simulink model "HEV_SeriesParallel"  (R2022b)
settings: Solver=ode23t  StartTime=0.0  StopTime=100  RelTol=0.0001  AbsTol=1e-05  EnableMultiTasking=on
PreLoadFcn:
  | load UrbanCycle1
  | load UrbanCycle2
  | load UrbanCycle3
  | load UrbanCycle4
  | load UrbanCycle5
  | 
  | assignin('base','decimation',1)
  | Pbatt = 21e3;
  | Vbatt =100;
  | Ts = 6e-5;   % time step
  | 
  | Drive_Cycle_Num = 1;
  | warning off Simulink:Commands:LoadMdlParameterizedLink
PostLoadFcn:
  | warning off Simulink:Engine:UsingDefaultMaxStepSize
  | warning off Simulink:blocks:MatchingGotoNotFound
  | warning off Simulink:blocks:MatchingFromNotFound
  | warning off Simulink:blocks:TDelayBufferTooSmall
  | warning off Simulink:SL_SaveWithParameterizedLinks_Warning
  | warning off Simulink:SL_TDelayBufferTooSmall
  | warning off Simulink:SL_OutputNotConnected
  | warning off Simulink:SL_SaveWithDisabledLinks_Warning
  | 
  | warning off Simulink:SL_SetParamLinkChangeWarn
  | 
  | warning('off','Simulink:SL_UINotUpdatedDuringRapidAccelSim');
  | warning off Simulink:Engine:OutputNotConnected
  | warning off Simulink:Engine:UINotUpdatedDuringRapidAccelSim
  | warning off Simulink:Engine:SaveWithParameterizedLinks_Warning
  | warning off Simulink:Engine:SolverMaskedZC
  | set_param('HEV_SeriesParallel','MaskedZcDiagnostic','none');
  | warning off Simulink:Engine:SolverInconsistentInitialConditionsWarnForDAE
  | set_param('HEV_SeriesParallel','IgnoredZcDiagnostic','none');
  | warning off Simulink:Engine:SolverIgnoredZCBracketing
  | set_param('HEV_SeriesParallel','MaxConsecutiveZCsMsg','none');
  | warning off Simulink:Engine:SolverConsecutiveZCNum
  | warning off Simulink:Engine:SolverMinStepSizeWarnForDAE
  | warning off Simulink:Engine:SolverMinStepNonlinearIterWarnForDAE
  | warning off simscape:compiler:sli:init:SolverNotRecommended
  | warning off Simulink:Commands:SetParamLinkChangeWarn
  | warning off xPCTarget:sampleTime:sampleTimeInvariance
  | warning off Simulink:blocks:TDelayFixedBuffer
  | 
  | warning('off','physmod:common:gl:sli:rtp:InvalidNonValueReference')
  | warning('off','physmod:common:gl:sli:rtp:InvalidNonValueReferenceMask')
  | 
  | Setup_HEV_Model_Configurations
  | 
  | % Commands to avoid warning at first run
  | % PS battery function
  | warning off MATLAB:illConditionedMatrix
  | try
  |    set_param(bdroot, 'SimulationCommand', 'update');
  | catch
  | end
  | warning on MATLAB:illConditionedMatrix
InitFcn:
  | Configure_HEV_Simulation
StartFcn:
  | tic;
StopFcn:
  | Elapsed_Sim_Time = toc; disp(['Elapsed time for ' bdroot ' = ' num2str(Elapsed_Sim_Time)])
model workspace (MAT data in the model file):
  guiH = 18054.0001221
undefined symbols (not defined in the file or in its folder): HEV_Param, sigbuilder_block
libraries: fl_lib x18, nesl_utility x11, HEV_Electrical_Lib x3, sdl_lib x2, HEV_Vehicle_Dynamics_Lib x2, simulink x1, spspowerguiLib x1
(part 1 of 2)
Description:
  | Hybrid Electric Vehicle, Series-Parallel
  | 
  | Copyright 2014-2022 The MathWorks(TM), Inc.
settings Model: ExtModeTrigDuration=200  TunableVars=Drive_Cycle_Num  TunableVarsStorageClass=Auto  Creator=tegel  LastModifiedBy=fedformi_new
settings SolverCC: AutoScaleAbsTol=off  ZcThreshold=0  ConsecutiveZCsStepRelTol=0.0001  ConcurrentTasks=on  ZeroCrossAlgorithm=Adaptive  AlgebraicLoopSolver=TrustRegion  PositivePriorityOrder=on
settings DataIOCC: SaveFormat=Array  SignalLoggingSaveFormat=ModelDataLogs  SignalLogging=off  DSMLogging=off  ReturnWorkspaceOutputs=off
settings OptimizationCC: BlockReduction=off  OptimizeBlockIOStorage=off  BufferReuse=off  GlobalBufferReuse=off  ExpressionFolding=off  ExpressionDepthLimit=2147483647  LocalBlockOutputs=off  ZeroExternalMemoryAtStartup=off  ZeroInternalMemoryAtStartup=off  InitFltsAndDblsToZero=on  EfficientMapNaN2IntZero=off  OptimizeDataStoreBuffers=off  BusAssignmentInplaceUpdate=off
settings DebuggingCC: AlgebraicLoopMsg=error  UnderspecifiedInitializationDetection=Classic  MergeDetectMultiDrivingBlocksExec=none  SignalResolutionControl=TryResolveAllWithWarning  MaxConsecutiveZCsMsg=none  MaskedZcDiagnostic=none  IgnoredZcDiagnostic=none  SigSpecEnsureSampleTimeMsg=none  FcnCallInpInsideContextMsg=warning  UnconnectedInputMsg=warning  UnconnectedOutputMsg=warning  UnconnectedLineMsg=warning  AllowSymbolicDim=off  UnknownTsInhSupMsg=none  StateNameClashWarn=warning  PregeneratedLibrarySubsystemCodeDiagnostic=none  SFUnexpectedBacktrackingDiag=warning  SFNoUnconditionalDefaultTransitionDiag=warning  SFExecutionAtInitializationDiag=none  SFMachineParentedDataDiag=warning  ArithmeticOperatorsInVariantConditions=warning
settings HardwareCC: TargetBitPerLong=64  TargetBitPerPointer=64  TargetBitPerSizeT=64  TargetBitPerPtrDiffT=64  TargetLongLongMode=on  TargetIntDivRoundTo=Zero  TargetEndianess=LittleEndian  TargetWordSize=64  TargetHWDeviceType=MATLAB Host
settings ModelReferenceCC: EnableRefExpFcnMdlSchedulingChecks=on  PropagateSignalLabelsOutOfModel=off
settings SFSimCC: SimUseLocalCustomCode=off  SimParseCustomCode=off  CustomCodeUndefinedFunction=UseInterfaceOnly
settings RTWCC: RTWUseLocalCustomCode=off  Toolchain=Simulink Real-Time Toolchain  BuildConfiguration=Faster Runs  TargetLang=C++  DLArmComputeVersion=19.05
settings CodeAppCC: StateflowObjectComments=on
settings GRTTargetCC: TargetLangStandard=C++03 (ISO)  CodeInterfacePackaging=C++ class
settings ConfigComp: CovMetricSettings=dw  CovSaveCumulativeToWorkspaceVar=on  CovSaveSingleToWorkspaceVar=on  CovExternalEMLEnable=off  CovSFcnEnable=off
settings SimscapeCC: ExplicitSolverDiagnosticOptions=none  SimscapeNormalizeSystem=off  SimscapeLogType=all  SimscapeLogName=simlog_HEVSP  SimscapeLogLimitData=off

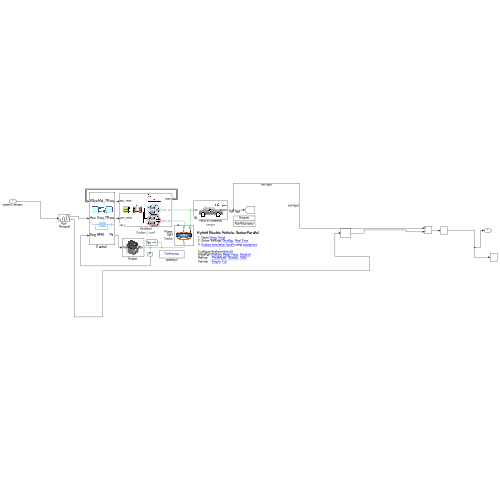
[thumbnail: Simulink's stored preview of the top-level diagram]
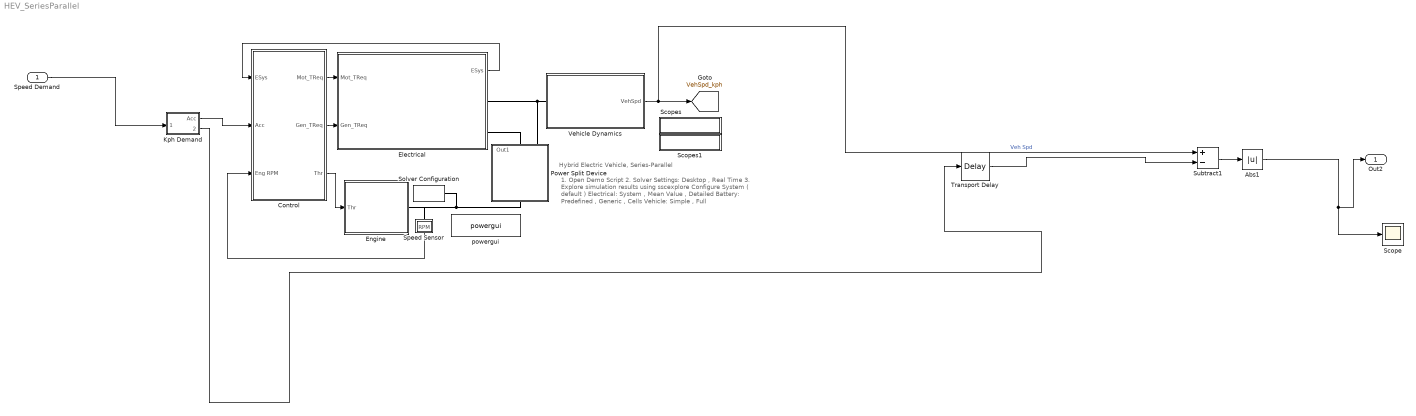
== system HEV_SeriesParallel ==
  note: 1. Open Demo Script
      | 2. Solver Settings: Desktop , Real Time
      | 3. Explore simulation results using sscexplore
      |
      | Configure System ( default )
      | Electrical: System , Mean Value , Detailed
      | Battery: Predefined , Generic , Cells
      | Vehicle: Simple , Full
  note: Hybrid Electric Vehicle, Series-Parallel
  Speed Demand : Inport
  Abs1 : Abs  SaturateOnIntegerOverflow=off
  Control : Subsystem
      mask Display:
      | image('HEV_Control_IMAGE.jpg');
      | port_label('input',1,'ESys');
      | port_label('input',2,'Acc');
      | port_label('input',3,'Eng RPM');
      | port_label('output',1,'Mot_TReq');
      | port_label('output',2,'Gen_TReq');
      | port_label('output',3,'Thr');
  Electrical : Subsystem  BlockChoice=System Level  Variant=on  VariantControlMode=label  LabelModeActiveChoice=System_Level  mask{popup_electricalvariant=System Level, popup_batteryvariantsystem=Predefined, popup_batteryvariantdetailed=Generic}
      mask prompts: popup_electricalvariant "Fidelity of Electrical System"; popup_batteryvariantsystem "Battery Model"; popup_batteryvariantdetailed "Battery Model"
      mask init:
      | if(popup_electricalvariant==1)
      |     set_param(gcb,'LabelModeActiveChoice','System_Level');
      |     set_param([gcb '/System Level'],'popup_batteryvariant',get_param(gcb,'popup_batteryvariantsystem'));
      | elseif(popup_electricalvariant==2)
      | 	set_param(gcb,'LabelModeActiveChoice','Mean_Value');
      |     set_param([gcb '/Mean Value'],'popup_batteryvariant',get_param(gcb,'popup_batteryvariantdetailed'));
      | elseif(popup_electricalvariant==3)
      |     set_param(gcb,'LabelModeActiveChoice','Detailed');
      |     set_param([gcb '/Detailed'],'popup_batteryvariant',get_param(gcb,'popup_batteryvariantdetailed'));
      | end
      | 
      | %blk = find_system(gcbh, 'FollowLinks','on','SearchDepth', 1, 'Parent', gcb, 'VariantObject', get_param(gcb,'activevariant'));
      settings: AttributesFormatString=%<ActiveVariant>
      mask TypeOptions popup_electricalvariant: System Level | Mean Value | Detailed
      mask Callback popup_electricalvariant:
      | maskObj = Simulink.Mask.get(gcb);
      | bas_h = maskObj.getParameter('popup_batteryvariantsystem');
      | bad_h = maskObj.getParameter('popup_batteryvariantdetailed');
      | if strcmp(get_param(gcb,'popup_electricalvariant'),'System Level')
      |     bas_h.Visible = 'on';
      |     bad_h.Visible = 'off';
      | else
      |     bas_h.Visible = 'off';
      |     bad_h.Visible = 'on';
      | end
      | clear maskObj
      mask TypeOptions popup_batteryvariantsystem: Predefined | Generic | Cells
      mask TypeOptions popup_batteryvariantdetailed: Predefined | Generic
      mask Display:
      | ele_var = get_param(gcb,'ActiveVariant');
      | batt_var = get_param([gcb '/' strrep(ele_var,'_',' ') '/Battery'],'ActiveVariant');
      | imagestr = ['HEV_Electrical_' strrep(ele_var,'_','') '_' batt_var '_IMAGE.jpg'];
      | image(imagestr);
  Engine : Subsystem  RequirementInfo={} %GIDa_8d15d6ea_be00_49db_a7ed_57a5c222ce3a
      mask Display:
      | image('HEV_Engine_IMAGE.jpg');
      | port_label('input',1,'Thr');
      | port_label('RConn',1,'Sh');
  Kph Demand : Subsystem
      mask Display:
      | plotstr=['UrbanCycle' evalin('base','num2str(Drive_Cycle_Num)')];
      | plot(evalin('base',[plotstr '.time']),evalin('base',[plotstr '.SpdKph']));
      | text(evalin('base',['0.7*max(' plotstr '.time)']),evalin('base',['0.25*max(' plotstr '.SpdKph)']),evalin('base','num2str(Drive_Cycle_Num)'));
  Power Split Device : Subsystem
      mask Display:
      | image('HEV_Planetary_Gear_IMAGE.jpg');
      | color('black');
      | port_label('Lconn',1,'C');
      | port_label('Rconn',1,'S');
      | port_label('Rconn',2,'R');
  Scope : Scope
  Scopes : Subsystem  mask(Data Acquisition){}
      mask Display: disp('Scopes');
  Scopes1 : Subsystem  mask(Data Acquisition){}
      mask Display: disp('Fuel Economy');
  Solver Configuration : nesl_utility/Solver Configuration  PhysicalDomain=network_engine_domain  SubClassName=solver  LeftPortType=input  RightPortType=generic  Tones=[]  Harmonics=[]  SimulateNoise=off  Profile=off  UseLocalSampling=off  EnableSwitchedLinearOptims=on  FrequencyDomain=off  UseCCode=off  RelTol=0.001  AbsTol=1e-06  MinStep=1e-09  ToWorkspace=off  RevertToSquareIcSolve=off  NumHomotopyIterations=100  PhasorMode=off  PhasorModeNumHarmonics=1  ConsistencySolver=NEWTON_FTOL  IndexReductionMethod=DerivativeReplacement  DoDC=off  ResidualTolerance=1e-8  ConsistencyTolSource=GLOBAL  ConsistencyAbsTol=0.001  ConsistencyRelTol=0.001  ConsistencyTolFactor=0.001  UseLocalSolver=off  LocalSolverChoice=NE_BACKWARD_EULER_ADVANCER  ResolveIndetEquations=on  FunctionEvalNumThread=1  LocalSolverSampleTime=0.005  DoFixedCost=off  MaxNonlinIter=3  MaxModeIter=2  ComputeImpulses=off  ImpulseIterations=2  LinearAlgebra=Sparse  LinearAlgebraNumThread=0  EquationFormulation=NE_TIME_EF  DelaysMemoryBudget=1024  AutomaticFiltering=on  FilteringTimeConstant=0.001  PartitionStorageMethod=AS_NEEDED  PartitionMemoryBudget=1024  PartitionMethod=FAST
  Speed Sensor : Subsystem
      mask Display: disp('S')
  Subtract1 : Sum  Inputs=+-
  Transport Delay : TransportDelay  DelayTime=0.7
  Vehicle Dynamics : Subsystem  BlockChoice=Simple  Variant=on  VariantControlMode=label  LabelModeActiveChoice=Simple
      settings: AttributesFormatString=%<ActiveVariant>
      mask Display:
      | blk = find_system(gcbh, 'SearchDepth', 1, 'Parent', gcb, 'VariantObject', get_param(gcb,'activevariant'));
      | eval(get_param(blk, 'MaskDisplay'));
  powergui : spspowerguiLib/powergui  SimulationMode=Continuous  SampleTime=Ts  frequency=60  Iterations=50  frequencyindice=0  Pbase=100e6  ErrMax=1e-4  UnitsV=kV  UnitsW=MW  buscounter=0  FunctionMessages=off  echomessages=off  EnableUseOfTLC=off  CurrentSourceSwitches=off  DisableSnubberDevices=off  DisableRonSwitches=off  DisableVfSwitches=off  DisplayEquations=off  AutomaticDiscreteSolvers=off  SolverType=Tustin  Interpol=off  ExternalGateDelay=off  methode=off  Ts=0  x0status=blocks  SPID=on  SwTol=0  HookPort=off  NonlinearTolerance=0  nMaxIteration=15  ContinueOnMaxIteration=off  RestoreLinks=warning  ResistiveCurrentMeasurement=off  Frange=[0:2:500]  Ylog=off  Xlog=on  ShowGrid=off  save=off  variable=ZData  structure=0  ZoomFFT=on  StartTime=0.0  cycles=1  DisplayStyle=1  fundamental=60  FreqAxis=off  MaxFrequency=1000  frequencyindicesteady=1  RmsSteady=1  display=off
  Out2 : Outport
  tag scope: VehSpd_kph=global
  wires:
  Speed Sensor/1(RPM) -> Control/3(Eng RPM)
  Control/1(Mot_TReq) -> Electrical/1(Mot_TReq)
  Control/2(Gen_TReq) -> Electrical/2(Gen_TReq)
  Control/3(Thr) -> Engine/1(Thr)
  Kph Demand/1(Acc) -> Control/2(Acc)
  Electrical/1(ESys) -> Control/1("ESys ")
  Vehicle Dynamics/1(VehSpd) -> Subtract1/1, [VehSpd_kph]  "Veh Spd"
  Abs1/1 -> Scope/1, Out2/1
  Subtract1/1 -> Abs1/1
  Kph Demand/2(DesiredVelocity) -> Transport Delay/1
  Transport Delay/1 -> Subtract1/2
  Speed Demand/1 -> Kph Demand/1(Speed Demand)
  connections:
  Electrical/RConn2 -- Power Split Device/RConn1
  Power Split Device/RConn2 -- Electrical/RConn1 -- Vehicle Dynamics/LConn1
  Speed Sensor/LConn1 -- Engine/RConn1 -- Power Split Device/LConn1 -- Solver Configuration/RConn1

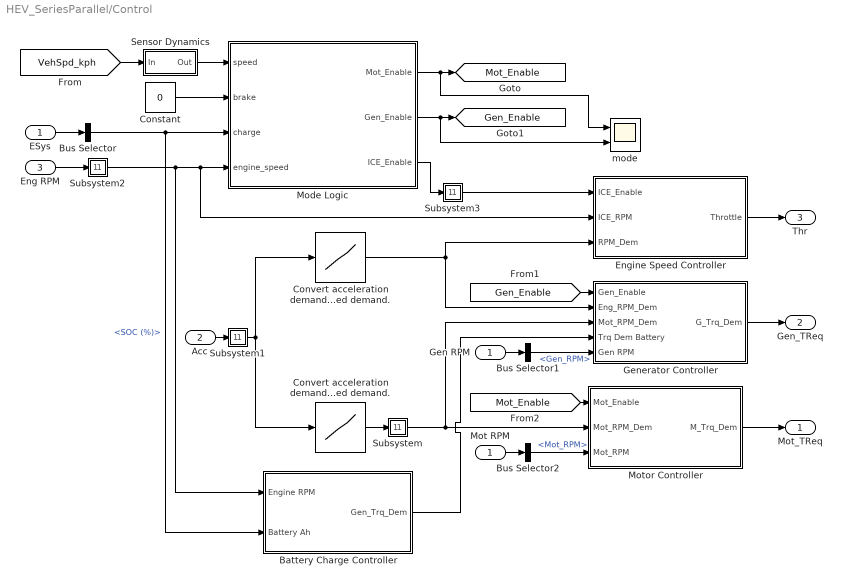
== system HEV_SeriesParallel/Control ==
  "ESys " : Inport
  Acc : Inport  Port=2
  Eng RPM : Inport  Port=3
  Battery Charge Controller : Subsystem
  Bus Selector : BusSelector  OutputSignals=Batt.SOC (%)
  Bus Selector1 : BusSelector  OutputSignals=Gen_RPM
  Bus Selector2 : BusSelector  OutputSignals=Mot_RPM
  Constant : Constant  Value=0
  Convert acceleration demand to engine speed demand. : Lookup  InputValues=[0 0.1 1]  Table=[0 800 4000]  SaturateOnIntegerOverflow=off
  Convert acceleration demand to motor speed demand. : Lookup  InputValues=[0 1]  Table=[0 2500]  SaturateOnIntegerOverflow=off
  Engine Speed Controller : Subsystem
  Gen RPM : InportShadow
  Generator Controller : Subsystem
  Mode Logic : Stateflow chart  TreatAsAtomicUnit=on
  Mot RPM : InportShadow
  Motor Controller : Subsystem
  Sensor Dynamics : Subsystem  mask(First-order lag supporting vector signals){b=HEV_Param.ICE.sensor_time_constant, x_initial=0}
      mask prompts: b "Filter time constant"; x_initial "Initial output"
      mask help: Models a lag of the form 1/(b*s+1) where s is the Laplace operator.
  Subsystem : Subsystem
      mask Display: disp('S')
  Subsystem1 : Subsystem
      mask Display: disp('S')
  Subsystem2 : Subsystem
      mask Display: disp('S')
  Subsystem3 : Subsystem
      mask Display: disp('S')
  mode : Scope  NumInputPorts=2
  Mot_TReq : Outport  VectorParamsAs1DForOutWhenUnconnected=off
  Gen_TReq : Outport  Port=2  VectorParamsAs1DForOutWhenUnconnected=off
  Thr : Outport  Port=3  VectorParamsAs1DForOutWhenUnconnected=off
  tag scope: Gen_Enable=global, Mot_Enable=global
  wires:
  Acc/1 -> Subsystem1/1(In1)
  Eng RPM/1 -> Subsystem2/1(In1)
  Engine Speed Controller/1(Throttle) -> Thr/1
  Convert acceleration demand to motor speed demand./1 -> Subsystem/1(In1)
  Convert acceleration demand to engine speed demand./1 -> Engine Speed Controller/3(RPM_Dem), Generator Controller/2(Eng_RPM_Dem)
  Bus Selector2/1 -> Motor Controller/3(Mot_RPM)  "<Mot_RPM>"
  Motor Controller/1(M_Trq_Dem) -> Mot_TReq/1
  Generator Controller/1(G_Trq_Dem) -> Gen_TReq/1
  "ESys "/1 -> Bus Selector/1
  Subsystem2/1(Eng_RPM_Meas) -> Battery Charge Controller/1(Engine RPM), Mode Logic/4(engine_speed), Engine Speed Controller/2(ICE_RPM)
  Bus Selector/1 -> Battery Charge Controller/2(Battery Ah), Mode Logic/3(charge)  "<SOC (%)>"
  Constant/1 -> Mode Logic/2(brake)
  Mode Logic/3(ICE_Enable) -> Subsystem3/1(In1)
  Subsystem3/1(Gen_RPM_Dem) -> Engine Speed Controller/1(ICE_Enable)
  Mode Logic/2(Gen_Enable) -> mode/2, [Gen_Enable]
  Mode Logic/1(Mot_Enable) -> mode/1, [Mot_Enable]
  Sensor Dynamics/1(Out) -> Mode Logic/1(speed)
  Bus Selector1/1 -> Generator Controller/5(Gen RPM)  "<Gen_RPM>"
  Subsystem/1(Motor_RPM_Dem) -> Motor Controller/2(Mot_RPM_Dem), Generator Controller/3(Mot_RPM_Dem)
  [Gen_Enable] -> Generator Controller/1(Gen_Enable)
  [Mot_Enable] -> Motor Controller/1(Mot_Enable)
  Battery Charge Controller/1(Gen_Trq_Dem) -> Generator Controller/4(Trq Dem Battery)
  Gen RPM/1 -> Bus Selector1/1
  Mot RPM/1 -> Bus Selector2/1
  Subsystem1/1(Accel) -> Convert acceleration demand to motor speed demand./1, Convert acceleration demand to engine speed demand./1
  [VehSpd_kph] -> Sensor Dynamics/1(In)

== system HEV_SeriesParallel/Electrical ==
  note: Variants of Electrical System
  Mot_TReq : Inport
  Gen_TReq : Inport  Port=2
  Detailed : HEV_Electrical_Lib/Detailed  VariantControl=Detailed  popup_batteryvariant=Predefined
      link override Battery: OverrideUsingVariant=Generic  LabelModeActiveChoice=Predefined
  Mean Value : HEV_Electrical_Lib/Mean Value  VariantControl=Mean_Value  popup_batteryvariant=Predefined
      link override Battery: OverrideUsingVariant=Generic  LabelModeActiveChoice=Predefined
  System Level : HEV_Electrical_Lib/System Level  VariantControl=System_Level  popup_batteryvariant=Predefined
      link override Battery: LabelModeActiveChoice=Generic
  Mot_Sh : PMIOPort  Side=Right
  Gen_Sh : PMIOPort  Port=2  Side=Right
  ESys : Outport  VectorParamsAs1DForOutWhenUnconnected=off

== system HEV_SeriesParallel/Engine ==
  Thr : Inport
  Engine Shaft Inertia : fl_lib/Mechanical/Rotational Elements/Inertia  inertia=HEV_Param.ICE.Shaft_Inertia kg*m^2  num_ports=foundation.enum.numPorts2.one  w_specify=on  w_priority=High  w=0 rad/s  w_nominal_specify=off  w_nominal_unit=rad/s  w_nominal_value=1  t_specify=off  t_priority=High  t=0 N*m  t_nominal_specify=off  t_nominal_unit=N*m  t_nominal_value=1
  Generic Engine : sdl_lib/Engines & Motors/Generic Engine  input_type=sdl.enum.GenericEngineInputType.NormalizedThrottle  model_parameterization=1  engine_type=1  Trq_max=380 N*m  w_Trq_max=4300 rpm  P_max=HEV_Param.ICE.Max_Power W  w_P_max=HEV_Param.ICE.Speed_At_Max_Power rpm  w_max=HEV_Param.ICE.Max_Speed rpm  w_min=500 rpm  w_tab=[ 500 1000 2e+3 3e+3 4e+3 5e+3 6e+3 7e+3 ] rpm  trq_tab=[ 380 380 380 380 350 280 200 80 ] N*m  pwr_tab=[ 2e+4 4e+4 7.8e+4 1.2e+5 1.45e+5 1.48e+5 1.25e+5 6e+4 ] W  interp_method=1  w_thr=100 rpm  model_inertia=0  inertia=1 kg*m^2  initial_velocity=800 rpm  model_time_constant=0  time_constant=0.2 s  initial_normalized_throttle=0  fc_model=1  fc_per_rev=25 mg/rev  fc_w_tab=[ 1000 2e+3 3e+3 4e+3 5e+3 6e+3 ] rpm  fc_trq_tab=[ 0 80 160 200 240 320 360 400 ] N*m  fc_tab=[ 0.5 0.9 1.4 1.6 1.9 2.7 3.4 4.4; 1 1.7 2.7 3.1 3.6 5 6 7.4; 1.4 2.7 4 4.8 5.6 7.5 8.5 10.5; 2 3.6 5.8 6.7 8 10.4 11.7 13.3; 2.5 4.8 7.9 9.4 10.8 14 16.2 18.6; 3.1 6 10.3 11.9 13.8 18.4 22 26.5 ] g/s  bmep_tab=[ 0 250 500 625 750 1000 1.15e+3 1.25e+3 ] kPa  bsfc_tab=[ 410 380 300 280 270 290 320 380; 410 370 290 270 260 270 285 320; 415 380 290 275 265 270 270 300; 420 390 310 290 285 280 280 285; 430 410 340 320 310 300 310 320; 450 430 370 340 330 330 350 380 ] g/hr/kW  fc_interp_method=1  displaced_volume=400 cm^3  rev_per_cycle=2  idle_speed=0  idle_speed_reference=1000 rpm  tau_controller=1 s  idle_w_thr=1 rpm  redline=0  redline_speed=5000 rpm  tau_redline=1 s  redline_w_thr=1 rpm
      settings: InternalSimscapePortConfiguration="{\"Bottom\":[],\"Left\":[{\"id\":\"ThrNorm\",\"label\":\"Thr\",\"type\":\"input\"},{\"id\":\"B\",\"label\":\"B\",\"type\":\"foundation.mechanical.rotational.rotational\"}],\"Right\":[{\"id\":\"P\",\"label\":\"P\",\"type\":\"output\"},{\"id\":\"FC\",\"label\":\"FC\",\"type\":\"output\"},{\"id\":\"F\",\"label\":\"F\",\"type\":\"foundation.mechanical.rotational.rotational\"}],\"Top\":[]}"
  MRRef Engine Housing : fl_lib/Mechanical/Rotational Elements/Mechanical Rotational Reference
  MRRef Engine Shaft : fl_lib/Mechanical/Rotational Elements/Mechanical Rotational Reference
  Rotational Damper : fl_lib/Mechanical/Rotational Elements/Rotational Damper  D=HEV_Param.ICE.Friction N*m/(rad/s)  w_specify=off  w_priority=High  w=0 rad/s  w_nominal_specify=off  w_nominal_unit=rad/s  w_nominal_value=1  t_specify=off  t_priority=High  t=0 N*m  t_nominal_specify=off  t_nominal_unit=N*m  t_nominal_value=1
  Sensor : Subsystem
      mask Display: disp('S');
  Simulink-PS Converter : nesl_utility/Simulink-PS Converter  PhysicalDomain=network_engine_domain  SubClassName=ps_input  LeftPortType=input  RightPortType=output  PseudoPeriodic=off  Frequencies=[]  NoiseDistribution=none  NoiseParameters=[]  Unit=1  AffineConversion=off  FilteringAndDerivatives=zero  SimscapeFilterOrder=1  InputFilterTimeConstant=0.005  UdotUserProvided=0
  Sh : PMIOPort  Side=Right
  wires:
  Thr/1 -> Simulink-PS Converter/1  "Throttle"
  connections:
  Sensor/RConn1 -- Sh/RConn1
  MRRef Engine Shaft/LConn1 -- Rotational Damper/RConn1
  Simulink-PS Converter/RConn1 -- Generic Engine/LConn1
  MRRef Engine Housing/LConn1 -- Generic Engine/LConn2
  Sensor/LConn1 -- Generic Engine/RConn3 -- Rotational Damper/LConn1 -- Engine Shaft Inertia/LConn1

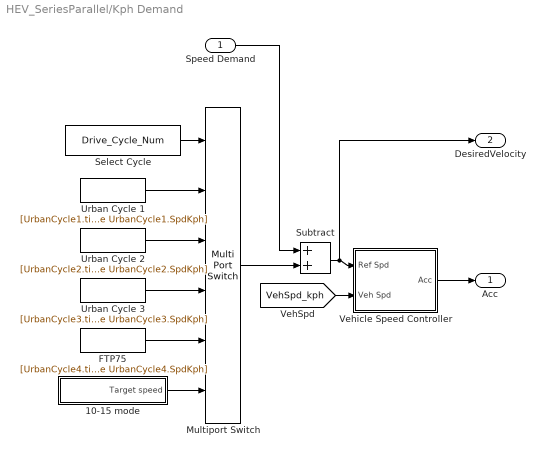
== system HEV_SeriesParallel/Kph Demand ==
  Speed Demand : Inport
  "10-15 mode " : Subsystem  Tag=STV Subsys  LoadFcn=sigbuilder_block('load');  StartFcn=sigbuilder_block('start');  StopFcn=sigbuilder_block('stop');  ClipboardFcn=sigbuilder_block('clipboard');  mask(Sigbuilder block){tuvar=[0:10]}
      mask help: Sigbuilder GUI
      mask init:
      | if ~strcmp(get_param(bdroot(gcbh),'SimulationStatus'),'stopped') tuvar = sigbuilder_block('maskInit'); end
      settings: CopyFcn=sigbuilder_block('copy');  DeleteFcn=sigbuilder_block('delete');  ModelCloseFcn=sigbuilder_block('modelClose');  PreSaveFcn=sigbuilder_block('preSave');  PauseFcn=sigbuilder_block('pause')  ContinueFcn=sigbuilder_block('continue')  NameChangeFcn=sigbuilder_block('namechange');  OpenFcn=sigbuilder_block('open',[561.6 178.2 550.8 399 ]);  CloseFcn=sigbuilder_block('close');
      mask Display: plot(0, 0, 100, 100,[2, 2, 32, 32, 2], [68, 8, 8, 68, 68],[32, 2], [38, 38], [32, 19, 2],[53, 60, 44], [32, 17, 17, 2],[16, 16, 31, 31]);txt = getActiveGroup(gcbh);text(2, 100, txt,'verticalAlignment', 'top');
  FTP75 : FromWorkspace  VariableName=[UrbanCycle4.time UrbanCycle4.SpdKph]
  Multiport Switch : MultiPortSwitch  Inputs=5  SaturateOnIntegerOverflow=off  InputSameDT=off
  Select Cycle : Constant  Value=Drive_Cycle_Num
  Subtract : Sum
  Urban Cycle 1 : FromWorkspace  VariableName=[UrbanCycle1.time UrbanCycle1.SpdKph]
  Urban Cycle 2 : FromWorkspace  VariableName=[UrbanCycle2.time UrbanCycle2.SpdKph]
  Urban Cycle 3 : FromWorkspace  VariableName=[UrbanCycle3.time UrbanCycle3.SpdKph]
  Vehicle Speed Controller : Subsystem
  Acc : Outport  VectorParamsAs1DForOutWhenUnconnected=off
  DesiredVelocity : Outport  Port=2  VectorParamsAs1DForOutWhenUnconnected=off
  wires:
  Urban Cycle 3/1 -> Multiport Switch/4
  Select Cycle/1 -> Multiport Switch/1
  Urban Cycle 2/1 -> Multiport Switch/3
  Urban Cycle 1/1 -> Multiport Switch/2
  Vehicle Speed Controller/1(Acc) -> Acc/1
  [VehSpd_kph] -> Vehicle Speed Controller/2(Veh Spd)
  FTP75/1 -> Multiport Switch/5
  "10-15 mode "/1(Target speed) -> Multiport Switch/6
  Speed Demand/1 -> Subtract/1
  Multiport Switch/1 -> Subtract/2
  Subtract/1 -> DesiredVelocity/1, Vehicle Speed Controller/1(Ref Spd)

== system HEV_SeriesParallel/Power Split Device ==
  note: For port placement
  Constant : Constant
  Planetary Gear : sdl_lib/Gears/Planetary Gear  rs_ratio=HEV_Param.Power_Split.Ratio_Ring2Sun  friction_model=2  efficiency=[ 0.96 0.98 ]  temperature_TLU=[ 280 300 320 ] K  efficiency_sp_TLU=[ 0.95 0.9 0.85 ]  efficiency_rp_TLU=[ 0.95 0.9 0.85 ]  pwr_thr=[ 0.001 0.001 ] W  mu_visc=[ 0.02 0 ] N*m/(rad/s)  model_inertia=0  planet_inertia=0.001 kg*m^2  thermal_mass=50 J/K  T_init=300 K
  Sensor Carrier Shaft : Subsystem
      mask Display: disp('S')
  Sensor Ring Shaft : Subsystem
      mask Display: disp('S')
  Sensor Sun Shaft : Subsystem
      mask Display: disp('S')
  S : PMIOPort  Side=Right
  R : PMIOPort  Port=2  Side=Right
  C : PMIOPort  Port=3  Side=Left
  Out1 : Outport  VectorParamsAs1DForOutWhenUnconnected=off
  wires:
  Constant/1 -> Out1/1
  connections:
  S/RConn1 -- Sensor Sun Shaft/RConn1
  Planetary Gear/RConn1 -- Sensor Ring Shaft/LConn1
  Planetary Gear/RConn2 -- Sensor Sun Shaft/LConn1
  R/RConn1 -- Sensor Ring Shaft/RConn1
  Sensor Carrier Shaft/LConn1 -- C/RConn1
  Sensor Carrier Shaft/RConn1 -- Planetary Gear/LConn1

== system HEV_SeriesParallel/Scopes ==
  Batt DCDC Scopes : Subsystem
  Car Scopes : Subsystem
  Demux1 : Demux  Outputs=2
  Drivetrain Scopes : Subsystem
  Electricals Scopes : Subsystem
  ICE Scopes : Subsystem
  Mode Logic : Subsystem
  Motor Generator Scopes : Subsystem
  wires:
  Electricals Scopes/1(V) -> Demux1/1

== system HEV_SeriesParallel/Scopes1 ==
  note: Fuel Economy
  (L/100 km) : Display
      settings: Decimation=decimation
  (MPG) : Display
      settings: Decimation=decimation
  (km/L) : Display
      settings: Decimation=decimation
  Calculate Fuel Economy : Subsystem
  Fuel Consumption Table : Lookup2D  RowIndex=HEV_Param.ICE.FC.Speed_Vector  ColumnIndex=HEV_Param.ICE.FC.Torque_Vector  Table=HEV_Param.ICE.FC.Consumption_Table  SaturateOnIntegerOverflow=off  InputSameDT=off
  Total Fuel Used (L) : Display
      settings: Decimation=decimation
  wires:
  Calculate Fuel Economy/1(Liter/100Km) -> (L/100 km)/1
  Calculate Fuel Economy/3(MPG) -> (MPG)/1
  [VehSpd_kph] -> Calculate Fuel Economy/1(Kph)
  Calculate Fuel Economy/4(Fuel Used (L)) -> Total Fuel Used (L)/1
  Calculate Fuel Economy/2(Km/Liter) -> (km/L)/1
  Fuel Consumption Table/1 -> Calculate Fuel Economy/2(Fuel Flow g/s)
  [engine_speed] -> Fuel Consumption Table/1
  [Carrier_Trq_Nm] -> Fuel Consumption Table/2

== system HEV_SeriesParallel/Speed Sensor ==
  Ideal Rotational Motion Sensor : fl_lib/Mechanical/Mechanical Sensors/Ideal Rotational Motion Sensor  reference=foundation.enum.MeasurementReference.difference  acceleration_port=false  velocity_port=true  position_port=true  wrap_angle=simscape.enum.onoff.off  offset=0 rad
  Mechanical Rotational Reference : fl_lib/Mechanical/Rotational Elements/Mechanical Rotational Reference
  PS-Simulink Converter1 : nesl_utility/PS-Simulink Converter  PhysicalDomain=network_engine_domain  SubClassName=ps_output  LeftPortType=input  RightPortType=output  PseudoPeriodic=off  Frequencies=[]  VectorFormat=1-D array  Unit=rpm  AffineConversion=off
  Sensor Dynamics : Subsystem  mask(First-order lag supporting vector signals){b=HEV_Param.ICE.sensor_time_constant, x_initial=0}
      mask prompts: b "Filter time constant"; x_initial "Initial output"
      mask help: Models a lag of the form 1/(b*s+1) where s is the Laplace operator.
  Shaft : PMIOPort  Side=Left
  RPM : Outport  VectorParamsAs1DForOutWhenUnconnected=off
  wires:
  PS-Simulink Converter1/1 -> Sensor Dynamics/1(In)
  Sensor Dynamics/1(Out) -> RPM/1
  connections:
  PS-Simulink Converter1/LConn1 -- Ideal Rotational Motion Sensor/RConn2
  Mechanical Rotational Reference/LConn1 -- Ideal Rotational Motion Sensor/RConn1
  Ideal Rotational Motion Sensor/LConn1 -- Shaft/RConn1

== system HEV_SeriesParallel/Vehicle Dynamics ==
  Full : HEV_Vehicle_Dynamics_Lib/Full  SystemSampleTime=-1  VariantControl=Full  VariantActivationTime=update diagram  Latency=0  AutoFrameSizeCalculation=off
  Simple : HEV_Vehicle_Dynamics_Lib/Simple  VariantControl=Simple  mass=HEV_Param.Vehicle.Mass  area=HEV_Param.Vehicle.Frontal_Area  Cd=HEV_Param.Vehicle.Aero_Drag_Coeff  radius=HEV_Param.Vehicle.Tire_Radius  wheel_inertia=HEV_Param.Vehicle.Wheel_Inertia  gear_ratio=HEV_Param.Vehicle.Engine_Vehicle_Gear_Ratio
  Sh : PMIOPort  Side=Left
  VehSpd : Outport  VectorParamsAs1DForOutWhenUnconnected=off

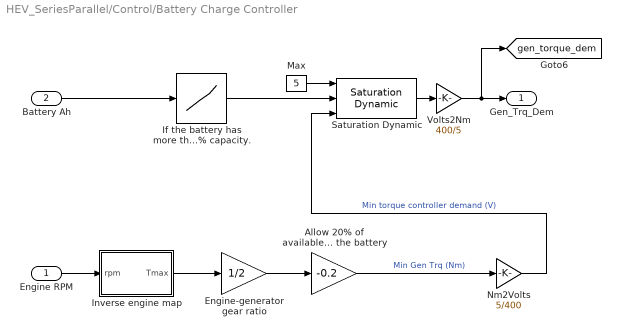
== system HEV_SeriesParallel/Control/Battery Charge Controller ==
  Engine RPM : Inport
  Battery Ah : Inport  Port=2
  Allow 20% of available torque to be used to charge the battery : Gain  Gain=-0.2
  Engine-generator gear ratio : Gain  Gain=1/2
  "If the battery has more than 100% rated capacity, then no generation is required. Linearly ramp to using 20% of engine torque for charging between 50% capacity and 100% capacity." : Lookup  InputValues=[0 50 100 150]  Table=[-5 -5 0 0]  SaturateOnIntegerOverflow=off
  Inverse engine map : Subsystem  mask(Inverse engine map){P0=43e3, rpm0=4000}
      mask prompts: P0 "Engine maximum power (W)"; rpm0 "Speed at maximum power (rpm)"
      mask help: Converts measured speed and demanded torque into normalized throttle demand. Assumes that the engine is modeled using the Simscape Driveline Generic Engine block with model parameterization set to Normalized 3rd-order polynomial matched to peak power.
      mask init:
      | w0 = 2*pi*rpm0/60;
  Max : Constant  Value=5
  Nm2Volts : Gain  Gain=5/400
  Saturation Dynamic : simulink/Discontinuities/Saturation Dynamic  OutMin=[]  OutMax=[]  OutDataTypeStr=Inherit: Same as second input  OutDataType=sfix(16)  OutScaling=2^-10  DoSatur=off
  Volts2Nm : Gain  Gain=400/5
  Gen_Trq_Dem : Outport  VectorParamsAs1DForOutWhenUnconnected=off
  tag scope: gen_torque_dem=global
  wires:
  Battery Ah/1 -> "If the battery has more than 100% rated capacity, then no generation is required. Linearly ramp to using 20% of engine torque for charging between 50% capacity and 100% capacity."/1
  Engine RPM/1 -> Inverse engine map/1(rpm)
  Inverse engine map/1(Tmax) -> Engine-generator gear ratio/1
  Allow 20% of available torque to be used to charge the battery/1 -> Nm2Volts/1  "Min Gen Trq (Nm)"
  Engine-generator gear ratio/1 -> Allow 20% of available torque to be used to charge the battery/1
  Nm2Volts/1 -> Saturation Dynamic/3  "Min torque controller demand (V)"
  Saturation Dynamic/1 -> Volts2Nm/1
  Max/1 -> Saturation Dynamic/1
  "If the battery has more than 100% rated capacity, then no generation is required. Linearly ramp to using 20% of engine torque for charging between 50% capacity and 100% capacity."/1 -> Saturation Dynamic/2
  Volts2Nm/1 -> Gen_Trq_Dem/1, [gen_torque_dem]

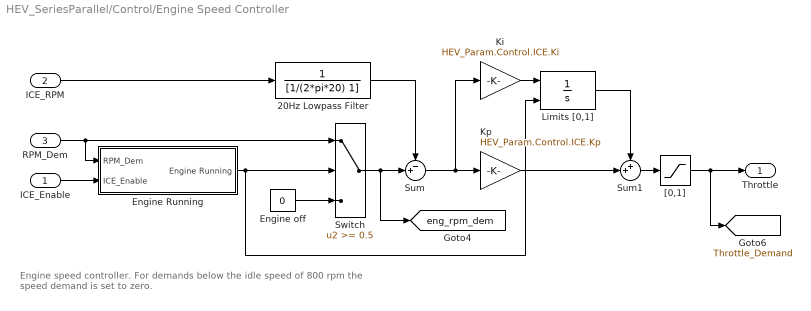
== system HEV_SeriesParallel/Control/Engine Speed Controller ==
  note: Engine speed controller. For demands below the idle speed of
      | 800 rpm the speed demand is set to zero.
  ICE_Enable : Inport
  ICE_RPM : Inport  Port=2
  RPM_Dem : Inport  Port=3
  20Hz Lowpass Filter : TransferFcn  Denominator=[1/(2*pi*20) 1]
  Engine Running : Subsystem
  Engine off : Constant  Value=0
  Ki : Gain  Gain=HEV_Param.Control.ICE.Ki
  Kp : Gain  Gain=HEV_Param.Control.ICE.Kp
  Limits [0,1] : Integrator  ExternalReset=either  LimitOutput=on  UpperSaturationLimit=1  LowerSaturationLimit=0
  Sum : Sum  Inputs=-+|
  Sum1 : Sum  Inputs=++|
  Switch : Switch  Threshold=0.5  SaturateOnIntegerOverflow=off  InputSameDT=off
  "[0,1]" : Saturate  UpperLimit=1  LowerLimit=0
  Throttle : Outport  VectorParamsAs1DForOutWhenUnconnected=off
  tag scope: Throttle_Demand=global, eng_rpm_dem=global
  wires:
  RPM_Dem/1 -> Switch/1, Engine Running/1(RPM_Dem)
  ICE_RPM/1 -> 20Hz Lowpass Filter/1
  Sum/1 -> Ki/1, Kp/1
  Ki/1 -> Limits [0,1]/1
  Kp/1 -> Sum1/2
  Limits [0,1]/1 -> Sum1/1
  20Hz Lowpass Filter/1 -> Sum/1
  Switch/1 -> Sum/2, [eng_rpm_dem]
  "[0,1]"/1 -> Throttle/1, [Throttle_Demand]
  Sum1/1 -> "[0,1]"/1
  Engine off/1 -> Switch/3
  ICE_Enable/1 -> Engine Running/2(ICE_Enable)
  Engine Running/1(Engine Running) -> Switch/2, Limits [0,1]/2

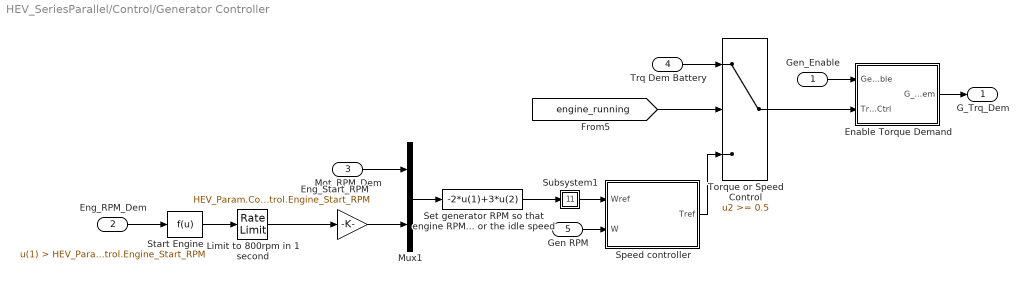
== system HEV_SeriesParallel/Control/Generator Controller ==
  Gen_Enable : Inport
  Eng_RPM_Dem : Inport  Port=2
  Mot_RPM_Dem : Inport  Port=3
  Trq Dem Battery : Inport  Port=4
  Gen RPM : Inport  Port=5
  Enable Torque Demand : Subsystem
  Eng_Start_RPM : Gain  Gain=HEV_Param.Control.Engine_Start_RPM
  Limit to 800rpm in 1 second : RateLimiter  SampleTimeMode=inherited
  Mux1 : Mux  Inputs=2
  Set generator RPM so that engine RPM is controlled to zero or the idle speed : Fcn  Expr=-2*u(1)+3*u(2)
  Speed controller : Subsystem
  Start Engine : Fcn  Expr=u(1) > HEV_Param.Control.Engine_Start_RPM
  Subsystem1 : Subsystem
      mask Display: disp('S')
  Torque or Speed Control : Switch  Threshold=0.5  SaturateOnIntegerOverflow=off  InputSameDT=off
  G_Trq_Dem : Outport  VectorParamsAs1DForOutWhenUnconnected=off
  wires:
  Set generator RPM so that engine RPM is controlled to zero or the idle speed/1 -> Subsystem1/1(In1)
  Mux1/1 -> Set generator RPM so that engine RPM is controlled to zero or the idle speed/1
  Limit to 800rpm in 1 second/1 -> Eng_Start_RPM/1
  Eng_Start_RPM/1 -> Mux1/2
  Gen RPM/1 -> Speed controller/2(W)
  Speed controller/1(Tref) -> Torque or Speed Control/3
  Subsystem1/1(Gen_RPM_Dem) -> Speed controller/1(Wref)
  Start Engine/1 -> Limit to 800rpm in 1 second/1
  Mot_RPM_Dem/1 -> Mux1/1
  Eng_RPM_Dem/1 -> Start Engine/1
  Trq Dem Battery/1 -> Torque or Speed Control/1
  Gen_Enable/1 -> Enable Torque Demand/1(Gen_Enable)
  [engine_running] -> Torque or Speed Control/2
  Enable Torque Demand/1(G_Trq_Dem) -> G_Trq_Dem/1
  Torque or Speed Control/1 -> Enable Torque Demand/2(TrqDemCtrl)

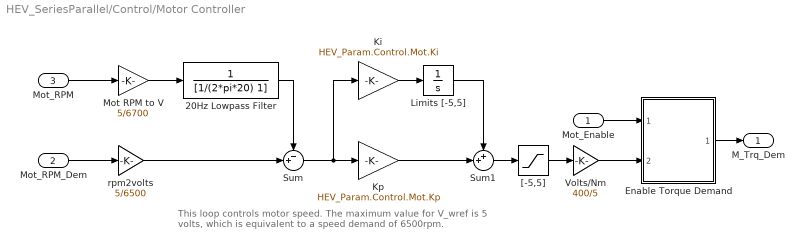
== system HEV_SeriesParallel/Control/Motor Controller ==
  note: This loop controls motor speed. The maximum value
      | for V_wref is 5 volts, which is equivalent to a speed
      | demand of 6500rpm.
  Mot_Enable : Inport
  Mot_RPM_Dem : Inport  Port=2
  Mot_RPM : Inport  Port=3
  20Hz Lowpass Filter : TransferFcn  Denominator=[1/(2*pi*20) 1]
  Enable Torque Demand : Subsystem
  Ki : Gain  Gain=HEV_Param.Control.Mot.Ki
  Kp : Gain  Gain=HEV_Param.Control.Mot.Kp
  Limits [-5,5] : Integrator  LimitOutput=on  UpperSaturationLimit=5  LowerSaturationLimit=-5
  Mot RPM to V : Gain  Gain=5/6700
  Sum : Sum  Inputs=-+|
  Sum1 : Sum  Inputs=++|
  Volts/Nm : Gain  Gain=400/5
  "[-5,5]" : Saturate  UpperLimit=5  LowerLimit=-5
  rpm2volts : Gain  Gain=5/6500
  M_Trq_Dem : Outport  VectorParamsAs1DForOutWhenUnconnected=off
  wires:
  "[-5,5]"/1 -> Volts/Nm/1
  Mot_RPM/1 -> Mot RPM to V/1
  Sum1/1 -> "[-5,5]"/1
  Sum/1 -> Ki/1, Kp/1
  Ki/1 -> Limits [-5,5]/1
  Kp/1 -> Sum1/2
  Limits [-5,5]/1 -> Sum1/1
  20Hz Lowpass Filter/1 -> Sum/1
  rpm2volts/1 -> Sum/2
  Mot RPM to V/1 -> 20Hz Lowpass Filter/1
  Volts/Nm/1 -> Enable Torque Demand/2(TrqDemCtrl)
  Mot_RPM_Dem/1 -> rpm2volts/1
  Mot_Enable/1 -> Enable Torque Demand/1(Mot_Enable)
  Enable Torque Demand/1(TrqDem) -> M_Trq_Dem/1

== system HEV_SeriesParallel/Control/Sensor Dynamics ==
  In : Inport
  Gain : Gain  Gain=1/b
  Integrator : Integrator  InitialCondition=x_initial
  Sum : Sum  Inputs=|+-  InputSameDT=on  SaturateOnIntegerOverflow=on  OutDataTypeStr=Inherit: Same as first input
  Out : Outport  VectorParamsAs1DForOutWhenUnconnected=off
  wires:
  Sum/1 -> Integrator/1
  In/1 -> Sum/1
  Integrator/1 -> Gain/1
  Gain/1 -> Sum/2, Out/1

== system HEV_SeriesParallel/Control/Subsystem ==
  In1 : Inport
  Motor_RPM_Dem : Outport  VectorParamsAs1DForOutWhenUnconnected=off
  tag scope: motor_rpm_dem=global
  wires:
  In1/1 -> [motor_rpm_dem], Motor_RPM_Dem/1

== system HEV_SeriesParallel/Control/Subsystem1 ==
  In1 : Inport
  Accel : Outport  VectorParamsAs1DForOutWhenUnconnected=off
  tag scope: Accelerator=global
  wires:
  In1/1 -> Accel/1, [Accelerator]

== system HEV_SeriesParallel/Control/Subsystem2 ==
  In1 : Inport
  Eng_RPM_Meas : Outport  VectorParamsAs1DForOutWhenUnconnected=off
  tag scope: eng_rpm_meas=global
  wires:
  In1/1 -> Eng_RPM_Meas/1, [eng_rpm_meas]

== system HEV_SeriesParallel/Control/Subsystem3 ==
  In1 : Inport
  Gen_RPM_Dem : Outport  VectorParamsAs1DForOutWhenUnconnected=off
  tag scope: ICE_Enable=global
  wires:
  In1/1 -> [ICE_Enable], Gen_RPM_Dem/1

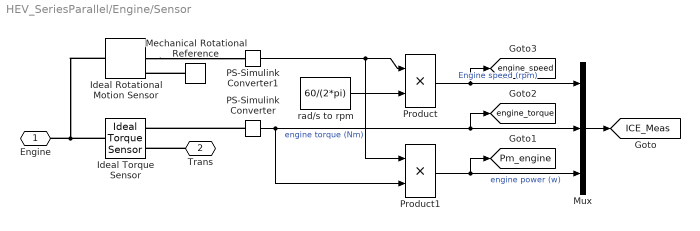
== system HEV_SeriesParallel/Engine/Sensor ==
  Ideal Rotational Motion Sensor : fl_lib/Mechanical/Mechanical Sensors/Ideal Rotational Motion Sensor  reference=foundation.enum.MeasurementReference.difference  acceleration_port=false  velocity_port=true  position_port=true  wrap_angle=simscape.enum.onoff.off  offset=0 rad
  Ideal Torque Sensor : fl_lib/Mechanical/Mechanical Sensors/Ideal Torque Sensor
  Mechanical Rotational Reference : fl_lib/Mechanical/Rotational Elements/Mechanical Rotational Reference
  Mux : Mux  Inputs=3
  PS-Simulink Converter : nesl_utility/PS-Simulink Converter  PhysicalDomain=network_engine_domain  SubClassName=ps_output  LeftPortType=input  RightPortType=output  PseudoPeriodic=off  Frequencies=[]  VectorFormat=1-D array  Unit=N*m  AffineConversion=off
  PS-Simulink Converter1 : nesl_utility/PS-Simulink Converter  PhysicalDomain=network_engine_domain  SubClassName=ps_output  LeftPortType=input  RightPortType=output  PseudoPeriodic=off  Frequencies=[]  VectorFormat=1-D array  Unit=rad/s  AffineConversion=off
  Product : Product  RndMeth=Zero
  Product1 : Product  RndMeth=Zero
  rad/s to rpm : Constant  Value=60/(2*pi)
  Engine : PMIOPort  Side=Left
  Trans : PMIOPort  Port=2  Side=Right
  tag scope: ICE_Meas=global, Pm_engine=global, engine_speed=global, engine_torque=global
  wires:
  PS-Simulink Converter/1 -> Product1/2, Mux/2, [engine_torque]  "engine torque (Nm)"
  Product1/1 -> Mux/3, [Pm_engine]  "engine power (w)"
  Product/1 -> Mux/1, [engine_speed]  "Engine speed (rpm)"
  PS-Simulink Converter1/1 -> Product/1, Product1/1
  rad/s to rpm/1 -> Product/2
  Mux/1 -> [ICE_Meas]
  connections:
  Ideal Torque Sensor/LConn1 -- Engine/RConn1 -- Ideal Rotational Motion Sensor/LConn1
  Trans/RConn1 -- Ideal Torque Sensor/RConn1
  PS-Simulink Converter/LConn1 -- Ideal Torque Sensor/RConn2
  Ideal Rotational Motion Sensor/RConn2 -- PS-Simulink Converter1/LConn1
  Mechanical Rotational Reference/LConn1 -- Ideal Rotational Motion Sensor/RConn1

== system HEV_SeriesParallel/Kph Demand/10-15 mode  ==
  Demux : Demux  Tag=STV Demux  Outputs=1
      settings: DisplayOption=none
  FromWs : FromWorkspace  Tag=STV FromWs  VariableName=tuvar
      SigBuilderData=|
      | common.afterFinalStr = 'Extrapolate'
      | common.sampleTime = '0'
      | dataSet.timeRange = [0 660]
      | dataSet.name = '10-15 Mode Cycle'
      | sbobj.Groups.Name = '10-15 Mode Cycle'
      | sbobj.Groups.Signals.Name = 'Target speed'
      | sbobj.Groups.Signals.XData = [0 44 51 66 73 89 103 118 128 130 142 152 159 179 186 201 208 224 238 253 263 265 277 287 294 314 321 336 343 359 373 388 398 400 412 422 429 494 512 524 528 532 548 558 569 579 589 593 615 620 640 650 660]
      | sbobj.Groups.Signals.YData = [0 0 20 20 0 0 40 40 20 20 40 20 0 0 20 20 0 0 40 40 20 20 40 20 0 0 20 20 0 0 40 40 20 20 40 20 0 0 50 50 40 40 60 60 70 70 50 50 70 70 30 0 0]
  Target speed : Outport  Tag=STV Outport  VectorParamsAs1DForOutWhenUnconnected=off
  wires:
  Demux/1 -> Target speed/1
  FromWs/1 -> Demux/1

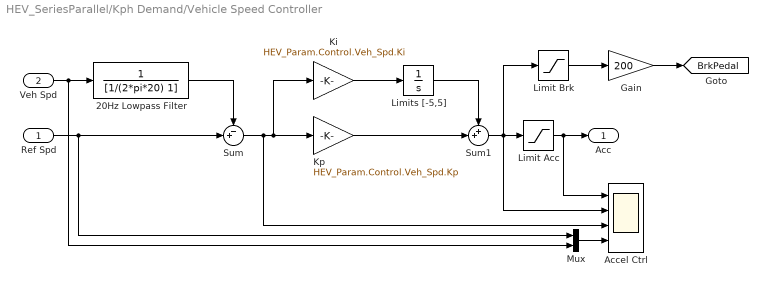
== system HEV_SeriesParallel/Kph Demand/Vehicle Speed Controller ==
  Ref Spd : Inport
  Veh Spd : Inport  Port=2
  20Hz Lowpass Filter : TransferFcn  Denominator=[1/(2*pi*20) 1]
  Accel Ctrl : Scope  NumInputPorts=4
  Gain : Gain  Gain=200
  Ki : Gain  Gain=HEV_Param.Control.Veh_Spd.Ki
  Kp : Gain  Gain=HEV_Param.Control.Veh_Spd.Kp
  Limit Acc : Saturate  UpperLimit=1  LowerLimit=0
  Limit Brk : Saturate  UpperLimit=0  LowerLimit=-inf
  Limits [-5,5] : Integrator  LimitOutput=on  UpperSaturationLimit=5  LowerSaturationLimit=-5
  Mux : Mux  Inputs=2
  Sum : Sum  Inputs=-+|
  Sum1 : Sum  Inputs=++|
  Acc : Outport  VectorParamsAs1DForOutWhenUnconnected=off
  tag scope: BrkPedal=global
  wires:
  Limit Acc/1 -> Acc/1, Accel Ctrl/1
  Ref Spd/1 -> Sum/2, Mux/1
  Veh Spd/1 -> 20Hz Lowpass Filter/1, Mux/2
  Sum1/1 -> Limit Brk/1, Limit Acc/1, Accel Ctrl/2
  Sum/1 -> Ki/1, Kp/1, Accel Ctrl/3
  Ki/1 -> Limits [-5,5]/1
  Kp/1 -> Sum1/2
  Limits [-5,5]/1 -> Sum1/1
  20Hz Lowpass Filter/1 -> Sum/1
  Mux/1 -> Accel Ctrl/4
  Limit Brk/1 -> Gain/1
  Gain/1 -> [BrkPedal]

== system HEV_SeriesParallel/Power Split Device/Sensor Carrier Shaft ==
  Ideal Rotational Motion Sensor : fl_lib/Mechanical/Mechanical Sensors/Ideal Rotational Motion Sensor  reference=foundation.enum.MeasurementReference.difference  acceleration_port=false  velocity_port=true  position_port=true  wrap_angle=simscape.enum.onoff.off  offset=0 rad
  Ideal Torque Sensor : fl_lib/Mechanical/Mechanical Sensors/Ideal Torque Sensor
  Mechanical Rotational Reference : fl_lib/Mechanical/Rotational Elements/Mechanical Rotational Reference
  PS-Simulink Converter : nesl_utility/PS-Simulink Converter  PhysicalDomain=network_engine_domain  SubClassName=ps_output  LeftPortType=input  RightPortType=output  PseudoPeriodic=off  Frequencies=[]  VectorFormat=1-D array  Unit=N*m  AffineConversion=off
  PS-Simulink Converter1 : nesl_utility/PS-Simulink Converter  PhysicalDomain=network_engine_domain  SubClassName=ps_output  LeftPortType=input  RightPortType=output  PseudoPeriodic=off  Frequencies=[]  VectorFormat=1-D array  Unit=rad/s  AffineConversion=off
  PG : PMIOPort  Side=Right
  Sh : PMIOPort  Port=2  Side=Left
  tag scope: Carrier_Spd_radps=global, Carrier_Trq_Nm=global
  wires:
  PS-Simulink Converter/1 -> [Carrier_Trq_Nm]  "Carrier torque (Nm)"
  PS-Simulink Converter1/1 -> [Carrier_Spd_radps]
  connections:
  PG/RConn1 -- Ideal Torque Sensor/RConn1 -- Ideal Rotational Motion Sensor/RConn1
  Mechanical Rotational Reference/LConn1 -- Ideal Rotational Motion Sensor/LConn1
  PS-Simulink Converter/LConn1 -- Ideal Torque Sensor/RConn2
  PS-Simulink Converter1/LConn1 -- Ideal Rotational Motion Sensor/RConn2
  Sh/RConn1 -- Ideal Torque Sensor/LConn1

== system HEV_SeriesParallel/Power Split Device/Sensor Ring Shaft ==
  Ideal Rotational Motion Sensor : fl_lib/Mechanical/Mechanical Sensors/Ideal Rotational Motion Sensor  reference=foundation.enum.MeasurementReference.difference  acceleration_port=false  velocity_port=true  position_port=true  wrap_angle=simscape.enum.onoff.off  offset=0 rad
  Ideal Torque Sensor : fl_lib/Mechanical/Mechanical Sensors/Ideal Torque Sensor
  Mechanical Rotational Reference : fl_lib/Mechanical/Rotational Elements/Mechanical Rotational Reference
  PS-Simulink Converter : nesl_utility/PS-Simulink Converter  PhysicalDomain=network_engine_domain  SubClassName=ps_output  LeftPortType=input  RightPortType=output  PseudoPeriodic=off  Frequencies=[]  VectorFormat=1-D array  Unit=N*m  AffineConversion=off
  PS-Simulink Converter1 : nesl_utility/PS-Simulink Converter  PhysicalDomain=network_engine_domain  SubClassName=ps_output  LeftPortType=input  RightPortType=output  PseudoPeriodic=off  Frequencies=[]  VectorFormat=1-D array  Unit=rad/s  AffineConversion=off
  PG : PMIOPort  Side=Right
  Sh : PMIOPort  Port=2  Side=Left
  tag scope: Ring_Spd_radps=global, Ring_Trq_Nm=global
  wires:
  PS-Simulink Converter/1 -> [Ring_Trq_Nm]  "Ring  torque (Nm)"
  PS-Simulink Converter1/1 -> [Ring_Spd_radps]  "Ring speed (rad/s)"
  connections:
  Ideal Rotational Motion Sensor/RConn1 -- PG/RConn1 -- Ideal Torque Sensor/RConn1
  Sh/RConn1 -- Ideal Torque Sensor/LConn1
  PS-Simulink Converter/LConn1 -- Ideal Torque Sensor/RConn2
  Mechanical Rotational Reference/LConn1 -- Ideal Rotational Motion Sensor/LConn1
  PS-Simulink Converter1/LConn1 -- Ideal Rotational Motion Sensor/RConn2

== system HEV_SeriesParallel/Power Split Device/Sensor Sun Shaft ==
  Ideal Rotational Motion Sensor : fl_lib/Mechanical/Mechanical Sensors/Ideal Rotational Motion Sensor  reference=foundation.enum.MeasurementReference.difference  acceleration_port=false  velocity_port=true  position_port=true  wrap_angle=simscape.enum.onoff.off  offset=0 rad
  Ideal Torque Sensor : fl_lib/Mechanical/Mechanical Sensors/Ideal Torque Sensor
  Mechanical Rotational Reference : fl_lib/Mechanical/Rotational Elements/Mechanical Rotational Reference
  PS-Simulink Converter : nesl_utility/PS-Simulink Converter  PhysicalDomain=network_engine_domain  SubClassName=ps_output  LeftPortType=input  RightPortType=output  PseudoPeriodic=off  Frequencies=[]  VectorFormat=1-D array  Unit=N*m  AffineConversion=off
  PS-Simulink Converter1 : nesl_utility/PS-Simulink Converter  PhysicalDomain=network_engine_domain  SubClassName=ps_output  LeftPortType=input  RightPortType=output  PseudoPeriodic=off  Frequencies=[]  VectorFormat=1-D array  Unit=rad/s  AffineConversion=off
  PG : PMIOPort  Side=Right
  Sh : PMIOPort  Port=2  Side=Left
  tag scope: Sun_Spd_radps=global, Sun_Trq_Nm=global
  wires:
  PS-Simulink Converter1/1 -> [Sun_Spd_radps]
  PS-Simulink Converter/1 -> [Sun_Trq_Nm]  "Sun_Trq_Nm"
  connections:
  Sh/RConn1 -- Ideal Torque Sensor/LConn1
  PS-Simulink Converter1/LConn1 -- Ideal Rotational Motion Sensor/RConn2
  PS-Simulink Converter/LConn1 -- Ideal Torque Sensor/RConn2
  Mechanical Rotational Reference/LConn1 -- Ideal Rotational Motion Sensor/LConn1
  PG/RConn1 -- Ideal Torque Sensor/RConn1 -- Ideal Rotational Motion Sensor/RConn1

== system HEV_SeriesParallel/Scopes/Batt DCDC Scopes ==
  DCDC Temp : Outport  VectorParamsAs1DForOutWhenUnconnected=off
  Batt Cell Temp : Outport  Port=2  VectorParamsAs1DForOutWhenUnconnected=off
  wires:
  [DCDC_SYS] -> DCDC Temp/1
  [Batt_Cell_Temp] -> Batt Cell Temp/1

== system HEV_SeriesParallel/Scopes/Car Scopes ==

== system HEV_SeriesParallel/Scopes/Drivetrain Scopes ==
  Mux6 : Mux  Inputs=2
  wires:
  [FA_RPM] -> Mux6/1
  [RA_RPM] -> Mux6/2

== system HEV_SeriesParallel/Scopes/Electricals Scopes ==
  Selector6 : Selector  InputPortWidth=8  IndexOptions=Index vector (dialog)  Indices=[1 2]  OutputSizes=1
  Selector7 : Selector  InputPortWidth=8  IndexOptions=Index vector (dialog)  Indices=[3 4]  OutputSizes=1
  Selector8 : Selector  InputPortWidth=8  IndexOptions=Index vector (dialog)  Indices=[5 6 7]  OutputSizes=1
  Selector9 : Selector  InputPortWidth=8  IndexOptions=Index vector (dialog)  Indices=[8]  OutputSizes=1
  V : Outport  VectorParamsAs1DForOutWhenUnconnected=off
  tag scope: SOC_out=global
  wires:
  Selector7/1 -> V/1  "Voltage (DC bus, Battery)"
  Selector9/1 -> [SOC_out]
  [Electricals] -> Selector8/1, Selector9/1, Selector7/1, Selector6/1

== system HEV_SeriesParallel/Scopes/ICE Scopes ==
  Demux : Demux  Outputs=3
  wires:
  [ICE_Meas] -> Demux/1

== system HEV_SeriesParallel/Scopes/Mode Logic ==
  Mux5 : Mux  Inputs=2
  wires:
  [ICE_Enable] -> Mux5/1
  [engine_running] -> Mux5/2

== system HEV_SeriesParallel/Scopes/Motor Generator Scopes ==
  Control Scopes : Subsystem
  Selector : Selector  InputPortWidth=4  IndexOptions=Index vector (dialog)  Indices=[1]  OutputSizes=1
  Selector1 : Selector  InputPortWidth=4  IndexOptions=Index vector (dialog)  Indices=[2]  OutputSizes=1
  Selector2 : Selector  InputPortWidth=4  IndexOptions=Index vector (dialog)  Indices=[3 4]  OutputSizes=1
  Selector3 : Selector  InputPortWidth=4  IndexOptions=Index vector (dialog)  Indices=[1]  OutputSizes=1
  Selector4 : Selector  InputPortWidth=4  IndexOptions=Index vector (dialog)  Indices=[2]  OutputSizes=1
  Selector5 : Selector  InputPortWidth=4  IndexOptions=Index vector (dialog)  Indices=[3 4]  OutputSizes=1
  M : Outport  VectorParamsAs1DForOutWhenUnconnected=off
  G : Outport  Port=2  VectorParamsAs1DForOutWhenUnconnected=off
  wires:
  Selector1/1 -> Control Scopes/1(In1), M/1  "Rotor speed (rpm)"
  [MotorDrive] -> Selector/1, Selector1/1, Selector2/1
  Selector4/1 -> Control Scopes/2(In2), G/1  "Rotor speed (rpm)"
  [GeneratorDrive] -> Selector5/1, Selector4/1, Selector3/1

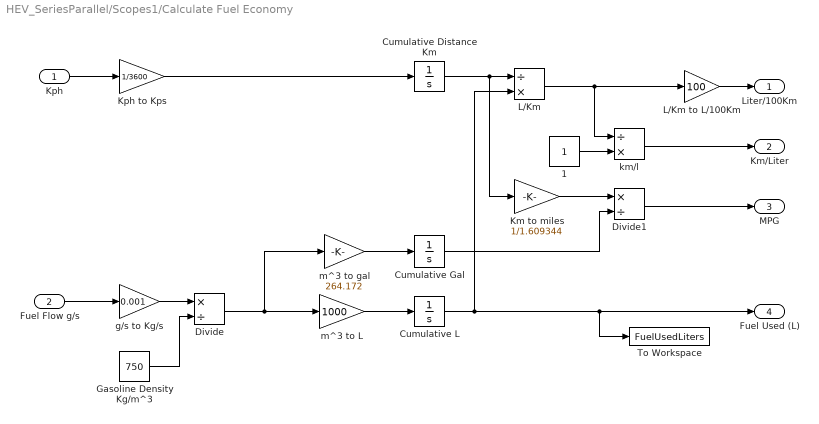
== system HEV_SeriesParallel/Scopes1/Calculate Fuel Economy ==
  Kph : Inport
  Fuel Flow g/s : Inport  Port=2
  1 : Constant
  Cumulative Distance Km : Integrator  InitialCondition=eps
  Cumulative Gal : Integrator  InitialCondition=eps
  Cumulative L : Integrator  InitialCondition=eps
  Divide : Product  Inputs=*/
  Divide1 : Product  Inputs=*/
  Gasoline Density Kg/m^3 : Constant  Value=750
  Km to miles : Gain  Gain=1/1.609344
  Kph to Kps : Gain  Gain=1/3600
  L/Km : Product  Inputs=/*
  L/Km to L/100Km : Gain  Gain=100
  To Workspace : ToWorkspace  VariableName=FuelUsedLiters  SampleTime=-1
      settings: MaxDataPoints=1
  g/s to Kg/s : Gain  Gain=0.001
  km/l : Product  Inputs=/*
  m^3 to L : Gain  Gain=1000
  m^3 to gal : Gain  Gain=264.172
  Liter/100Km : Outport  VectorParamsAs1DForOutWhenUnconnected=off
  Km/Liter : Outport  Port=2  VectorParamsAs1DForOutWhenUnconnected=off
  MPG : Outport  Port=3  VectorParamsAs1DForOutWhenUnconnected=off
  Fuel Used (L) : Outport  Port=4  VectorParamsAs1DForOutWhenUnconnected=off
  wires:
  km/l/1 -> Km/Liter/1
  1/1 -> km/l/2
  Divide1/1 -> MPG/1
  L/Km to L/100Km/1 -> Liter/100Km/1
  Fuel Flow g/s/1 -> g/s to Kg/s/1
  Kph/1 -> Kph to Kps/1
  Cumulative Gal/1 -> Divide1/2
  Km to miles/1 -> Divide1/1
  L/Km/1 -> km/l/1, L/Km to L/100Km/1
  Cumulative Distance Km/1 -> Km to miles/1, L/Km/1
  Cumulative L/1 -> L/Km/2, Fuel Used (L)/1, To Workspace/1
  Kph to Kps/1 -> Cumulative Distance Km/1
  m^3 to gal/1 -> Cumulative Gal/1
  m^3 to L/1 -> Cumulative L/1
  Divide/1 -> m^3 to gal/1, m^3 to L/1
  Gasoline Density Kg/m^3/1 -> Divide/2
  g/s to Kg/s/1 -> Divide/1

== system HEV_SeriesParallel/Speed Sensor/Sensor Dynamics ==
  In : Inport
  Gain : Gain  Gain=1/b
  Integrator : Integrator  InitialCondition=x_initial
  Sum : Sum  Inputs=|+-  InputSameDT=on  SaturateOnIntegerOverflow=on  OutDataTypeStr=Inherit: Same as first input
  Out : Outport  VectorParamsAs1DForOutWhenUnconnected=off
  wires:
  Sum/1 -> Integrator/1
  In/1 -> Sum/1
  Integrator/1 -> Gain/1
  Gain/1 -> Sum/2, Out/1

== system HEV_SeriesParallel/Control/Battery Charge Controller/Inverse engine map ==
  rpm : Inport
  Product : Product  InputSameDT=on  SaturateOnIntegerOverflow=on  OutDataTypeStr=Inherit: Same as first input
  Product1 : Product  Inputs=3  InputSameDT=on  SaturateOnIntegerOverflow=on  OutDataTypeStr=Inherit: Same as first input
  Sum1 : Sum  Inputs=|++  InputSameDT=on  SaturateOnIntegerOverflow=on  OutDataTypeStr=Inherit: Same as first input
  Sum2 : Sum  Inputs=|+-  InputSameDT=on  SaturateOnIntegerOverflow=on  OutDataTypeStr=Inherit: Same as first input
  p1 : Constant  Value=P0/w0
  p2 : Constant  Value=P0/w0^2
  p3 : Constant  Value=P0/w0^3
  rpm2rad/s : Gain  Gain=2*pi/60  SaturateOnIntegerOverflow=on  OutDataTypeStr=Inherit: Same as input  ParamDataTypeStr=Inherit: Same as input
  Tmax : Outport  VectorParamsAs1DForOutWhenUnconnected=off
  wires:
  p1/1 -> Sum1/1
  Sum2/1 -> Tmax/1  "Tmax"
  Product1/1 -> Sum2/2
  Sum1/1 -> Sum2/1
  p3/1 -> Product1/3
  Product/1 -> Sum1/2
  p2/1 -> Product/2
  rpm2rad/s/1 -> Product1/2, Product1/1, Product/1
  rpm/1 -> rpm2rad/s/1

== system HEV_SeriesParallel/Control/Engine Speed Controller/Engine Running ==
  RPM_Dem : Inport
  ICE_Enable : Inport  Port=2
  Alternate Logic : Subsystem
  Select Logic : ManualSwitch
  Engine Running : Outport  VectorParamsAs1DForOutWhenUnconnected=off
  tag scope: engine_running=global
  wires:
  RPM_Dem/1 -> Alternate Logic/1(RPM Dem)
  ICE_Enable/1 -> Select Logic/2
  Alternate Logic/1(ICE Enable) -> Select Logic/1
  Select Logic/1 -> Engine Running/1, [engine_running]
